simulink model "planGlobal_ros"  (R2024a)
settings: Solver=VariableStepAuto  StartTime=0.0  StopTime=10.0  RelTol=1e-3
InitFcn:
  | % Make sure server is running
  | svrMdlName = 'globalPlanServer';
  | load_system(svrMdlName);
  | set_param(svrMdlName,'SimulationCommand','Start');
  | pause(1);
StopFcn:
  | % Make sure server is running
  | svrMdlName = 'globalPlanServer';
  | load_system(svrMdlName);
  | set_param(svrMdlName,'SimulationCommand','Stop');
undefined symbols (not defined in the file): dem, goal, gridLoc, start, tuneableTerrainAwareParams, worldRes
libraries: roshelperlib x4, ros2lib x2, simulink x1
settings Model: Creator=cstabile  LastModifiedBy=cstabile

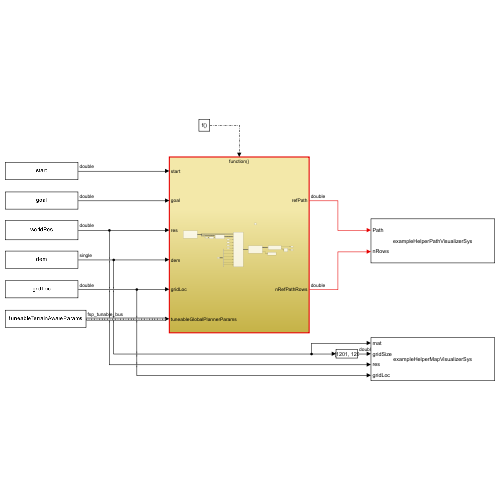
[thumbnail: Simulink's stored preview of the top-level diagram]
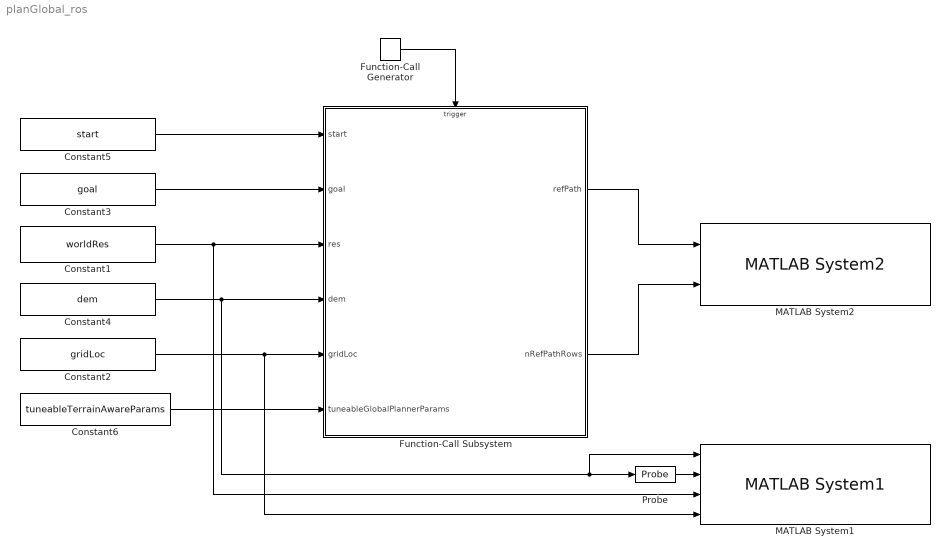
== system planGlobal_ros ==
  Constant1 : Constant  Value=worldRes
  Constant2 : Constant  Value=gridLoc
  Constant3 : Constant  Value=goal
  Constant4 : Constant  Value=dem
  Constant5 : Constant  Value=start
  Constant6 : Constant  Value=tuneableTerrainAwareParams  OutDataTypeStr=Bus: fsp_tunable_bus
  Function-Call Generator : simulink/Ports & Subsystems/Function-Call Generator  sample_time=1  numberOfIterations=1  DisallowWideOutput=off
  Function-Call Subsystem : Subsystem  TreatAsAtomicUnit=on
  MATLAB System1 : roshelperlib/MATLAB System1  MapType=Generic  DisplayVisual=on  SimulateUsing=Interpreted execution
  MATLAB System2 : roshelperlib/MATLAB System2  VisualizationParameters={'k-'}  PlotType=Line  DisplayVisual=on  SimulateUsing=Interpreted execution
  Probe : Probe  ProbeWidth=off  ProbeSampleTime=off  ProbeComplexSignal=off  ProbeSignalDimensions=on
  wires:
  Constant1/1 -> MATLAB System1/3, Function-Call Subsystem/3(res)
  Probe/1 -> MATLAB System1/2
  Constant6/1 -> Function-Call Subsystem/6(tuneableGlobalPlannerParams)
  Constant3/1 -> Function-Call Subsystem/2(goal)
  Constant2/1 -> MATLAB System1/4, Function-Call Subsystem/5(gridLoc)
  Constant4/1 -> MATLAB System1/1, Probe/1, Function-Call Subsystem/4(dem)
  Function-Call Generator/1 -> Function-Call Subsystem/Trigger
  Function-Call Subsystem/1(refPath) -> MATLAB System2/1
  Function-Call Subsystem/2(nRefPathRows) -> MATLAB System2/2
  Constant5/1 -> Function-Call Subsystem/1(start)

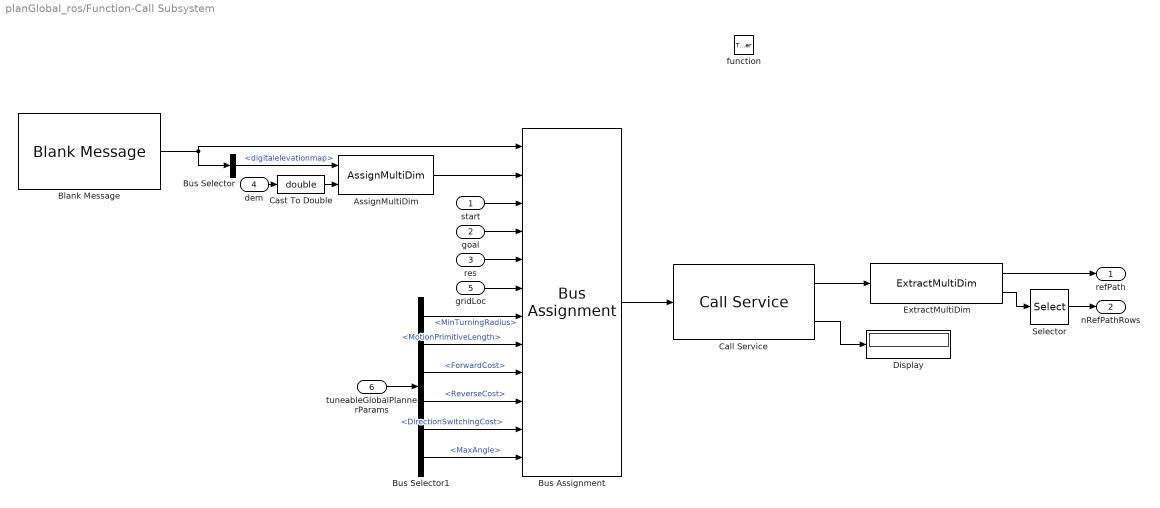
== system planGlobal_ros/Function-Call Subsystem ==
  start : Inport
  goal : Inport  Port=2
  res : Inport  Port=3
  dem : Inport  Port=4
  gridLoc : Inport  Port=5
  tuneableGlobalPlannerParams : Inport  Port=6  OutDataTypeStr=Bus: fsp_tunable_bus
  function : TriggerPort  TriggerType=function-call  VariantControl=(inherit)
  AssignMultiDim : roshelperlib/AssignMultiDim  SystemSampleTime=-1  VariantActivationTime=update diagram  AllowFlexibleInterface=on  Latency=0  AutoFrameSizeCalculation=off
  Blank Message : ros2lib/Blank Message  messageClass=Service Request  entityType=offroad_msg/PlanGlobal  messageType=offroad_msg/PlanGlobalRequest  SampleTime=inf
  Bus Assignment : BusAssignment  AssignedSignals=digitalelevationmap,start,goal,resolution,gridloc,tuneableterrainawareparams.minturningradius,tuneableterrainawareparams.motionprimitivelength,tuneableterrainawareparams.forwardcost,tuneableterrainawareparams.reversecost,tuneableterrainawareparams.directionswitchingcost,tuneableterrainawareparams.maxangle
  Bus Selector : BusSelector  OutputSignals=digitalelevationmap
  Bus Selector1 : BusSelector  OutputSignals=MinTurningRadius,MotionPrimitiveLength,ForwardCost,ReverseCost,DirectionSwitchingCost,MaxAngle
  Call Service : ros2lib/Call Service  topicSource=Specify your own  service=/planGlobal  serviceType=offroad_msg/PlanGlobal  connectionTimeout=10  ShowErrorCodeOutput=on  legacyBusStruct=off  QOSHistory=Keep last  QOSDepth=1  QOSReliability=Reliable  QOSDurability=Volatile  QOSDeadline=Inf  QOSLifespan=Inf  QOSLiveliness=Automatic  QOSLeaseDuration=Inf  QOSAvoidROSNamespaceConventions=off
  Cast To Double : DataTypeConversion  OutDataTypeStr=double  SaturateOnIntegerOverflow=off  RndMeth=Floor
  Display : Display
  ExtractMultiDim : roshelperlib/ExtractMultiDim  userDataType=double  dims=[1e4 3]  isVarsize=on  varsizeDims=[1 0]  returnFixedTF=on
  Selector : Selector  InputPortWidth=2  IndexOptions=Index vector (dialog)  Indices=1  OutputSizes=1
  refPath : Outport
  nRefPathRows : Outport  Port=2
  wires:
  Selector/1 -> nRefPathRows/1
  Call Service/1 -> ExtractMultiDim/1
  Blank Message/1 -> Bus Assignment/1, Bus Selector/1
  Bus Selector/1 -> AssignMultiDim/1  "<digitalelevationmap>"
  tuneableGlobalPlannerParams/1 -> Bus Selector1/1
  Bus Assignment/1 -> Call Service/1
  Call Service/2 -> Display/1
  ExtractMultiDim/1 -> refPath/1
  ExtractMultiDim/2 -> Selector/1
  dem/1 -> Cast To Double/1
  AssignMultiDim/1 -> Bus Assignment/2
  start/1 -> Bus Assignment/3
  goal/1 -> Bus Assignment/4
  res/1 -> Bus Assignment/5
  gridLoc/1 -> Bus Assignment/6
  Bus Selector1/6 -> Bus Assignment/12  "<MaxAngle>"
  Bus Selector1/5 -> Bus Assignment/11  "<DirectionSwitchingCost>"
  Bus Selector1/4 -> Bus Assignment/10  "<ReverseCost>"
  Bus Selector1/3 -> Bus Assignment/9  "<ForwardCost>"
  Bus Selector1/2 -> Bus Assignment/8  "<MotionPrimitiveLength>"
  Bus Selector1/1 -> Bus Assignment/7  "<MinTurningRadius>"
  Cast To Double/1 -> AssignMultiDim/2
